simulink model "A1_Inverter_sim"  (R2022b)
settings: Solver=ode23t  StartTime=0.0  StopTime=Tsim  MaxStep=Tstep  RelTol=1e-3  EnableMultiTasking=on
values from neighbouring files (symbols this model uses):
  A = sys_d.A    [A1_Inverter.m]    (also in a_invert.m = [0,       -R/L; control_b_a_1.m = [0 ,     -R/L)
  B = sys_d.B    [A1_Inverter.m]
  CL = 1    [A1_Inverter.m]
  Co = 5e-6    (= 5e-06)    [A1_Inverter.m]
  F = place(A,B,sfc_poles)    [A1_Inverter.m]
  L = place(A',C',obs_poles)'    [A1_Inverter.m]
  l = 2.5e-3    (= 0.0025)    [A1_Inverter.m]
  noise = 1    [A1_Inverter.m]
  obs = 1    [A1_Inverter.m]
  Ro = 0.1    [A1_Inverter.m]
  Tc = 1/fc    (= 0.0001)    [A1_Inverter.m]
  Ts = 1/fs    (= 5e-05)    [A1_Inverter.m]
  Tstep = Ts/100    (= 5e-07)    [A1_Inverter.m]
  Vdc = 100    [A1_Inverter.m]
undefined symbols (not defined in the file or in its folder): R, r
libraries: spsIGBTDiodeLib x4, spsSeriesRLCBranchLib x3, spsVoltageMeasurementLib x2, spsCurrentMeasurementLib x2, spsDCVoltageSourceLib x1, spsGroundLib x1, sps_lib x1, simulink x1
settings Model: Creator=Ricardo  LastModifiedBy=lucie
settings SolverCC: AlgebraicLoopSolver=TrustRegion
settings DataIOCC: LimitDataPoints=on  SaveFormat=Array  ReturnWorkspaceOutputs=off
settings OptimizationCC: LifeSpan=inf
settings DebuggingCC: SolverPrmCheckMsg=warning  UnconnectedInputMsg=warning  UnconnectedOutputMsg=warning  UnconnectedLineMsg=warning  SFUnexpectedBacktrackingDiag=warning  SFNoUnconditionalDefaultTransitionDiag=warning  SFExecutionAtInitializationDiag=none  SFMachineParentedDataDiag=warning  ArithmeticOperatorsInVariantConditions=warning
settings HardwareCC: ProdBitPerPointer=32  ProdBitPerSizeT=32  ProdBitPerPtrDiffT=32  ProdLargestAtomicFloat=None  ProdIntDivRoundTo=Undefined  ProdEndianess=Unspecified  ProdWordSize=32  ProdHWDeviceType=32-bit Generic
settings ModelReferenceCC: EnableRefExpFcnMdlSchedulingChecks=on  PropagateSignalLabelsOutOfModel=off
settings SFSimCC: SimUseLocalCustomCode=off  CustomCodeUndefinedFunction=UseInterfaceOnly
settings RTWCC: RTWUseLocalCustomCode=off  DLArmComputeVersion=19.05
settings CodeAppCC: StateflowObjectComments=on
settings GRTTargetCC: TargetLangStandard=C89/C90 (ANSI)
settings ConfigComp: CovMetricSettings=dw  CovSaveCumulativeToWorkspaceVar=on  CovSaveSingleToWorkspaceVar=on  CovExternalEMLEnable=off  CovSFcnEnable=off
settings SimscapeCC: SimscapeNormalizeSystem=off

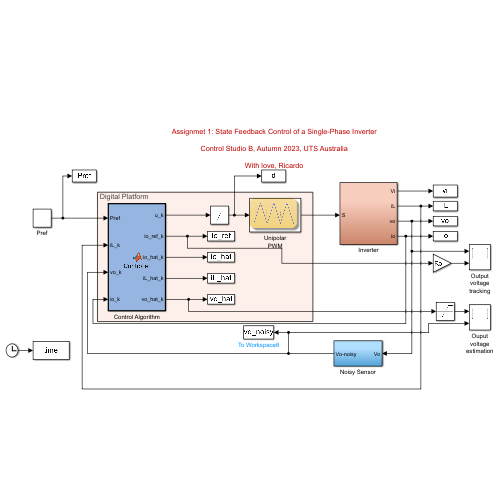
[thumbnail: Simulink's stored preview of the top-level diagram]
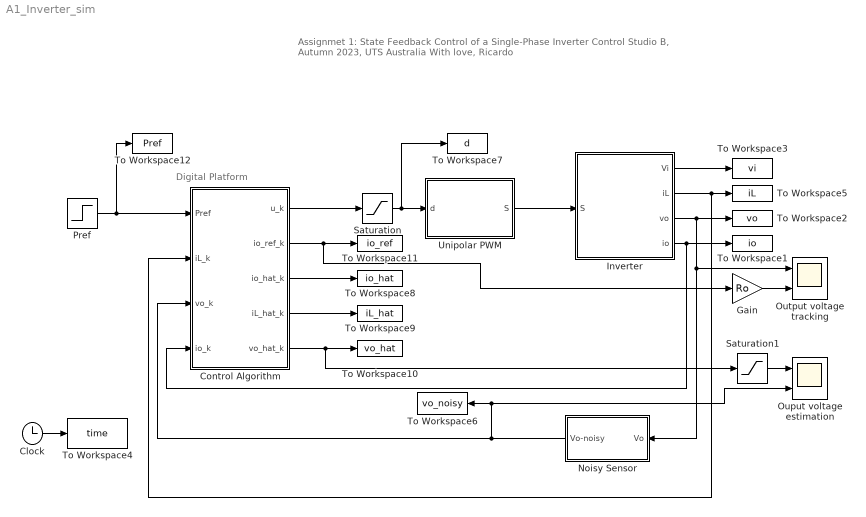
== system A1_Inverter_sim ==
  note: Digital Platform
  note: Assignmet 1: State Feedback Control of a Single-Phase Inverter
      |
      | Control Studio B, Autumn 2023, UTS Australia
      |
      | With love, Ricardo
  Clock : Clock
  Control Algorithm : MATLAB Function  TreatAsAtomicUnit=on  SystemSampleTime=Ts
  Gain : Gain  Gain=Ro
  Inverter : Subsystem
  Noisy Sensor : Subsystem
  Ouput voltage estimation : Scope  NumInputPorts=2
  Output voltage tracking : Scope  NumInputPorts=2
  Pref : Step  Time=0.04  Before=125  After=500  SampleTime=0
  Saturation : Saturate  UpperLimit=1  LowerLimit=-1
  Saturation1 : Saturate  UpperLimit=80  LowerLimit=-80
  To Workspace1 : ToWorkspace  VariableName=io  SampleTime=Tstep
  To Workspace10 : ToWorkspace  VariableName=vo_hat  SampleTime=Tstep
  To Workspace11 : ToWorkspace  VariableName=io_ref  SampleTime=Tstep
  To Workspace12 : ToWorkspace  VariableName=Pref  SampleTime=Tstep
  To Workspace2 : ToWorkspace  VariableName=vo  SampleTime=Tstep
  To Workspace3 : ToWorkspace  VariableName=vi  SampleTime=Tstep
  To Workspace4 : ToWorkspace  VariableName=time  SampleTime=Tstep
  To Workspace5 : ToWorkspace  VariableName=iL  SampleTime=Tstep
  To Workspace6 : ToWorkspace  VariableName=vo_noisy  SampleTime=Tstep
  To Workspace7 : ToWorkspace  VariableName=d  SampleTime=Tstep
  To Workspace8 : ToWorkspace  VariableName=io_hat  SampleTime=Tstep
  To Workspace9 : ToWorkspace  VariableName=iL_hat  SampleTime=Tstep
  Unipolar PWM : Subsystem
      mask Display: image('$imagefile'); % Use "Edit Image" on toolstrip to change.
  wires:
  Clock/1 -> To Workspace4/1
  Unipolar PWM/1(S) -> Inverter/1(S)
  Inverter/4(io) -> Control Algorithm/4(io_k), To Workspace1/1
  Inverter/3(vo) -> Output voltage tracking/1, Noisy Sensor/1(Vo), To Workspace2/1
  Inverter/2(iL) -> Control Algorithm/2(iL_k), To Workspace5/1
  Control Algorithm/1(u_k) -> Saturation/1
  Inverter/1(Vi) -> To Workspace3/1
  Saturation/1 -> To Workspace7/1, Unipolar PWM/1(d)
  Control Algorithm/2(io_ref_k) -> Gain/1, To Workspace11/1
  Control Algorithm/3(io_hat_k) -> To Workspace8/1
  Control Algorithm/4(iL_hat_k) -> To Workspace9/1
  Pref/1 -> To Workspace12/1, Control Algorithm/1(Pref)
  Control Algorithm/5(vo_hat_k) -> Saturation1/1, To Workspace10/1
  Noisy Sensor/1(Vo-noisy) -> Ouput voltage estimation/2, To Workspace6/1, Control Algorithm/3(vo_k)
  Saturation1/1 -> Ouput voltage estimation/1
  Gain/1 -> Output voltage tracking/2

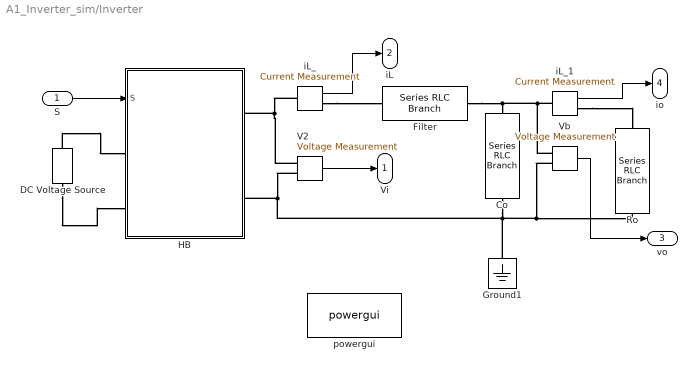
== system A1_Inverter_sim/Inverter ==
  S : Inport
  Co : spsSeriesRLCBranchLib/Series RLC Branch  LConnTagsString=__new0  RConnTagsString=__new0  BranchType=C  Resistance=R  Inductance=L  SetiL0=on  InitialCurrent=0  Capacitance=Co  Setx0=off  InitialVoltage=0  Measurements=Branch current
  DC Voltage Source : spsDCVoltageSourceLib/DC Voltage Source  Amplitude=Vdc  Measurements=None
  Filter : spsSeriesRLCBranchLib/Series RLC Branch  LConnTagsString=__new0  RConnTagsString=__new0  BranchType=L  Resistance=r  Inductance=l  SetiL0=on  InitialCurrent=0  Capacitance=1e-6  Setx0=off  InitialVoltage=0  Measurements=Branch current
  Ground1 : spsGroundLib/Ground  LConnTagsString=a
  HB : Subsystem
      mask Display: image('$imagefile'); % Use "Edit Image" on toolstrip to change.
  Ro : spsSeriesRLCBranchLib/Series RLC Branch  LConnTagsString=__new0  RConnTagsString=__new0  BranchType=R  Resistance=Ro  Inductance=L  SetiL0=on  InitialCurrent=0  Capacitance=1e-6  Setx0=off  InitialVoltage=0  Measurements=Branch current
  V2 : spsVoltageMeasurementLib/Voltage Measurement  Tag=PoWeRsYsTeMmEaSuReMeNt  PhasorSimulation=off  OutputType=Magnitude  PSBequivalent=0
  Vb : spsVoltageMeasurementLib/Voltage Measurement  Tag=PoWeRsYsTeMmEaSuReMeNt  PhasorSimulation=off  OutputType=Magnitude  PSBequivalent=0
  iL_ : spsCurrentMeasurementLib/Current Measurement  PhasorSimulation=off  OutputType=Complex  PSBequivalent=0
  iL_1 : spsCurrentMeasurementLib/Current Measurement  PhasorSimulation=off  OutputType=Complex  PSBequivalent=0
  powergui : sps_lib/powergui  SimulationMode=Discrete  SampleTime=Tstep  frequency=60  Iterations=50  frequencyindice=0  Pbase=100e6  ErrMax=1e-4  UnitsV=kV  UnitsW=MW  buscounter=0  FunctionMessages=off  echomessages=off  EnableUseOfTLC=off  CurrentSourceSwitches=off  DisableSnubberDevices=off  DisableRonSwitches=off  DisableVfSwitches=off  DisplayEquations=off  AutomaticDiscreteSolvers=off  SolverType=Tustin/Backward Euler (TBE)  Interpol=off  ExternalGateDelay=off  methode=off  Ts=0  x0status=blocks  SPID=off  SwTol=0  HookPort=off  NonlinearTolerance=1e-4  nMaxIteration=100  ContinueOnMaxIteration=off  RestoreLinks=warning  ResistiveCurrentMeasurement=off  Frange=[0:2:500]  Ylog=off  Xlog=on  ShowGrid=off  save=off  variable=ZData  structure=Currents  ZoomFFT=off  StartTime=0.0  cycles=2  DisplayStyle=4  fundamental=50  FreqAxis=off  MaxFrequency=2500  frequencyindicesteady=1  RmsSteady=1  display=off
  Vi : Outport
  iL : Outport  Port=2
  vo : Outport  Port=3
  io : Outport  Port=4
  wires:
  Vb/1 -> vo/1
  S/1 -> HB/1(S)
  V2/1 -> Vi/1
  iL_/1 -> iL/1
  iL_1/1 -> io/1
  connections:
  DC Voltage Source/RConn1 -- HB/LConn1
  Filter/RConn1 -- Vb/LConn1 -- iL_1/LConn1 -- Co/LConn1
  V2/LConn1 -- iL_/LConn1 -- HB/RConn1
  V2/LConn2 -- Vb/LConn2 -- Ro/RConn1 -- Ground1/LConn1 -- Co/RConn1 -- HB/RConn2
  DC Voltage Source/LConn1 -- HB/LConn2
  iL_/RConn1 -- Filter/LConn1
  iL_1/RConn1 -- Ro/LConn1

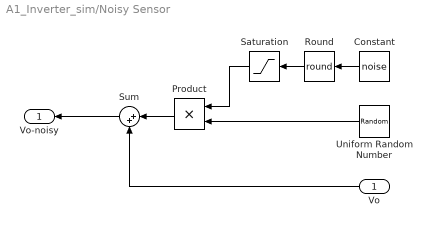
== system A1_Inverter_sim/Noisy Sensor ==
  Vo : Inport
  Constant : Constant  Value=noise
  Product : Product
  Round : Rounding  Operator=round
  Saturation : Saturate  UpperLimit=1  LowerLimit=0
  Sum : Sum  Inputs=|++
  Uniform Random Number : UniformRandomNumber  Seed=1  SampleTime=Tstep
  Vo-noisy : Outport
  wires:
  Vo/1 -> Sum/2
  Sum/1 -> Vo-noisy/1
  Product/1 -> Sum/1
  Uniform Random Number/1 -> Product/2
  Saturation/1 -> Product/1
  Constant/1 -> Round/1
  Round/1 -> Saturation/1

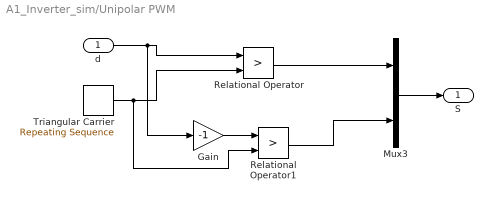
== system A1_Inverter_sim/Unipolar PWM ==
  d : Inport
  Gain : Gain  Gain=-1
  Mux3 : Mux  Inputs=2
  Relational Operator : RelationalOperator  Operator=>  OutDataTypeStr=boolean  RndMeth=Simplest
  Relational Operator1 : RelationalOperator  Operator=>  OutDataTypeStr=boolean  RndMeth=Simplest
  Triangular Carrier : simulink/Sources/Repeating Sequence  rep_seq_t=[0 Tc/2 Tc]  rep_seq_y=[-1 1 -1]
  S : Outport
  wires:
  Mux3/1 -> S/1
  d/1 -> Gain/1, Relational Operator/1
  Triangular Carrier/1 -> Relational Operator1/2, Relational Operator/2
  Gain/1 -> Relational Operator1/1
  Relational Operator/1 -> Mux3/1
  Relational Operator1/1 -> Mux3/2

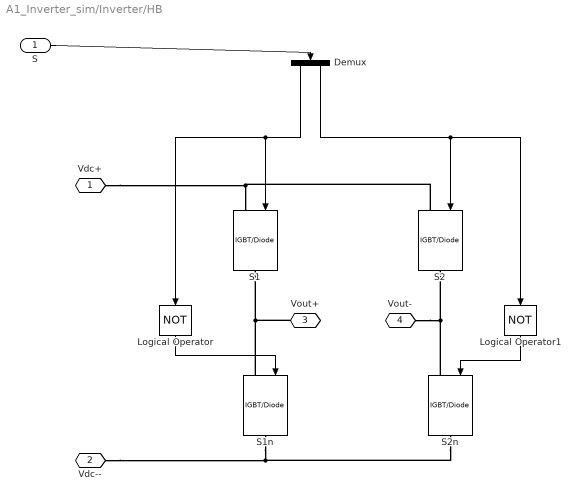
== system A1_Inverter_sim/Inverter/HB ==
  S : Inport
  Demux : Demux  Outputs=2
  Logical Operator : Logic  Operator=NOT  AllPortsSameDT=off  OutDataTypeStr=boolean
  Logical Operator1 : Logic  Operator=NOT  AllPortsSameDT=off  OutDataTypeStr=boolean
  S1 : spsIGBTDiodeLib/IGBT//Diode  Ron=1e-3  Rs=1e5  Cs=inf  Measurements=off
  S1n : spsIGBTDiodeLib/IGBT//Diode  Ron=1e-3  Rs=1e5  Cs=inf  Measurements=off
  S2 : spsIGBTDiodeLib/IGBT//Diode  Ron=1e-3  Rs=1e5  Cs=inf  Measurements=off
  S2n : spsIGBTDiodeLib/IGBT//Diode  Ron=1e-3  Rs=1e5  Cs=inf  Measurements=off
  Vdc+ : PMIOPort  Side=Left
  Vdc-- : PMIOPort  Port=2  Side=Left
  Vout+ : PMIOPort  Port=3  Side=Right
  Vout- : PMIOPort  Port=4  Side=Right
  wires:
  Logical Operator/1 -> S1n/1
  S/1 -> Demux/1
  Demux/1 -> Logical Operator/1, S1/1
  Logical Operator1/1 -> S2n/1
  Demux/2 -> Logical Operator1/1, S2/1
  connections:
  S1n/RConn1 -- Vdc--/RConn1 -- S2n/RConn1
  S1n/LConn1 -- Vout+/RConn1 -- S1/RConn1
  S2n/LConn1 -- Vout-/RConn1 -- S2/RConn1
  S2/LConn1 -- Vdc+/RConn1 -- S1/LConn1

== matlab function A1_Inverter_sim/Control Algorithm ==
  data: u_k output; io_ref_k output; io_hat_k output; iL_hat_k output; Pref input; iL_k input; vo_k input; io_k input; F parameter; Ts parameter; obs parameter; CL parameter; vo_hat_k output; l parameter; Vdc parameter; Ro parameter; Co parameter; A parameter; B parameter; L parameter
%% This function will provide the control action to be applied to system.
%  Also, this function will provide the instantaneous current reference
%  and the state estimates from the observer

% ***Check the script for possible Easter Eggs!!!
%%
function [u_k,io_ref_k,io_hat_k,iL_hat_k,vo_hat_k] = Controller(Pref,iL_k, vo_k, io_k, F, Ts, obs, CL, l, Vdc, Ro, Co, A, B, L)
%% Memory
persistent theta_k  % theta(k) = w*t(k)
if isempty(theta_k)
    theta_k = 0;
end
persistent x_hat_k 
if isempty(x_hat_k)
    x_hat_k = [5 10]'; %observer initialization x_hat(0) 
end

%% Measurements
x_k = [iL_k io_k]'; % measured system states

%% Reference Calculation
%  obtain Iref from Pref


%even though the power across the resistor is the only thing considered the
%current will lag behind the voltage after the reactive element
% determine impedance of the inductor
Xl = l*2*pi*50;
% Determine the difference between the resistive and reactive elements
phi = atan(Xl/Ro);
%magnitude of resistance
Z = sqrt(Ro^2 + Xl^2);

% Power output accounts for the real component of power only so convert
% accordingly
Iref = sqrt(2*Pref/(Z*cos(phi)));

io_ref_k = Iref*cos(theta_k);    %instantaneous current reference
iL_ref_k = io_ref_k;


%  obtain the reference vector xref_k from ioref_k
xref_k = [iL_ref_k io_ref_k]'; %state reference

%  obtain uref_k from iL_ref_k.
%  tip: for uref_k consider this form 
%       uref_k = a*cos(theta_k)+b*sin(theta_k);
%  then, obtain a and b
a=Iref*Ro/Vdc;
b=Iref*Ro^2*Co/Vdc;
uref_k=a*cos(theta_k)+b*sin(theta_k);
%% State Feedback Controller
if (CL==0)
    u_k = uref_k;  %Open-loop by applying uss
else
    %implement here your SFC
    if (obs~=1)
        u_k = -F*(x_k-xref_k)+uref_k;     %SFC without observer
    else
        u_k = -F*(x_hat_k-xref_k)+uref_k; %SFC with observer
    end
end

%% Observer 
% estimates to go out of this function (check these are correct)
io_hat_k = x_hat_k(2);
vo_hat_k = Ro*x_hat_k(2);
iL_hat_k = x_hat_k(1);

% Implement here your observer
x_hat_k = A*x_hat_k +B*u_k +L*(vo_k-vo_hat_k);

%% Updates (do not change this)
Dtheta = pi*Ts/10e-3; % for 50hz
theta_k = theta_k + Dtheta; %theta(k+1) = theta(k)+Dtheta;
if (theta_k>2*pi)
    theta_k = theta_k - 2*pi; %keep theta \in [0,2*pi]
end


end
